simulink model "car_suspension_absolutedisplacements_BumpStops"  (R2024a)
settings: Solver=VariableStepAuto  StartTime=0.0  StopTime=5  RelTol=1e-3
values from neighbouring files (symbols this model uses):
  C1 = 800    [axle_params.mat]    (also in suspension_params.mat; task1.m = 700; task2.m; task3.m)
  C2 = 3000    [axle_params.mat]    (also in suspension_params.mat = 6000; task1.m = 1500; task2.m = 1500; task3.m = C2_vals(j))
  C3 = 200    [axle_params.mat]    (also in suspension_params.mat; task2.m; task3.m; task4.m)
  K1 = 2000    [axle_params.mat]    (also in suspension_params.mat; task1.m = 2200; task2.m; task3.m)
  K2 = 30000    [axle_params.mat]    (also in suspension_params.mat = 50000; task1.m = 13000; task2.m = 13000; task3.m = K2_vals(i))
  K3 = 100000    [axle_params.mat]    (also in suspension_params.mat; task1.m = 120000; task2.m; task3.m)
  M1 = 60    [axle_params.mat]    (also in suspension_params.mat; task1.m = 50; task2.m; task3.m)
  M2 = 250    [axle_params.mat]    (also in suspension_params.mat; task1.m; task2.m; task3.m)
  M3 = 100    [axle_params.mat]    (also in suspension_params.mat; task1.m; task2.m; task3.m)
settings Model: Creator=co1il  LastModifiedBy=Alex
settings SolverCC: AlgebraicLoopSolver=TrustRegion
settings DataIOCC: ReturnWorkspaceOutputs=off
settings DebuggingCC: UnconnectedInputMsg=warning  UnconnectedOutputMsg=warning  UnconnectedLineMsg=warning  PregeneratedLibrarySubsystemCodeDiagnostic=none  ArithmeticOperatorsInVariantConditions=warning
settings ModelReferenceCC: EnableRefExpFcnMdlSchedulingChecks=on
settings SFSimCC: SimUseLocalCustomCode=off  CustomCodeUndefinedFunction=UseInterfaceOnly
settings RTWCC: RTWUseLocalCustomCode=off  GPUComputeCapability=3.5
settings CodeAppCC: StateflowObjectComments=on

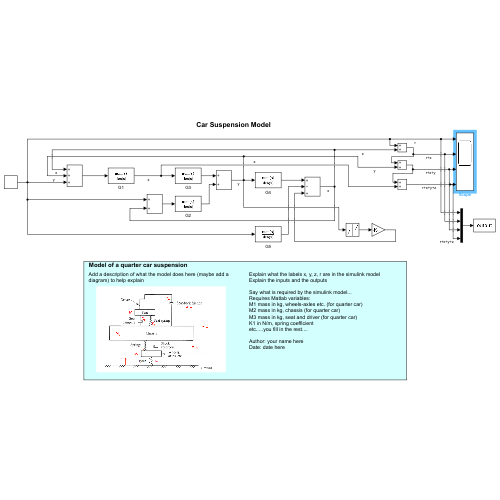
[thumbnail: Simulink's stored preview of the top-level diagram]
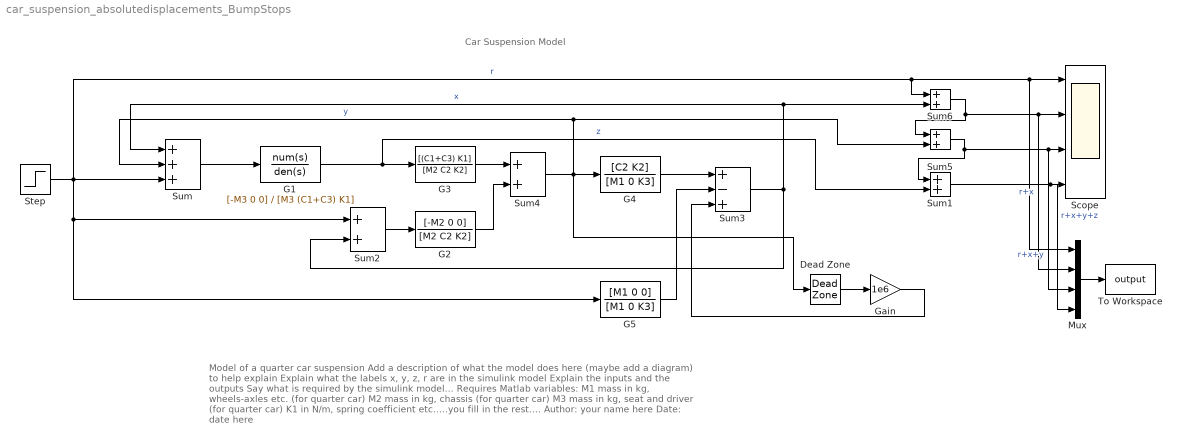
== system car_suspension_absolutedisplacements_BumpStops ==
  note: Model of a quarter car suspension
      |
      | Add a description of what the model does here (maybe add a diagram) to help explain
      |
      | Explain what the labels x, y, z, r are in the simulink model
      | Explain the inputs and the outputs
      |
      | Say what is required by the simulink model...
      | Requires Matlab variables:
      | M1 mass in kg, wheels-axles etc. (for quarter car)
      | M2 mass in kg, chassis (for quarter car)
      | M3 mass in kg, seat and driver (for quarter car)
      | K1 in N/m, spring coefficient
      | etc.....you fill in the rest....
      |
      | Author: your name here
      | Date: date here
  note: Car Suspension Model
  Dead Zone : DeadZone  LowerValue=-0.02  UpperValue=0.02
  G1 : TransferFcn  Numerator=[-M3 0 0]  Denominator=[M3 (C1+C3) K1]
  G2 : TransferFcn  Numerator=[-M2 0 0]  Denominator=[M2 C2 K2]
  G3 : TransferFcn  Numerator=[(C1+C3) K1]  Denominator=[M2 C2 K2]
  G4 : TransferFcn  Numerator=[C2 K2]  Denominator=[M1 0 K3]
  G5 : TransferFcn  Numerator=[M1 0 0]  Denominator=[M1 0 K3]
  Gain : Gain  Gain=1e6
  Mux : Mux
  Scope : Scope  NumInputPorts=4
  Step : Step  After=0.1  SampleTime=0
  Sum : Sum  Inputs=+++
  Sum{1..2,4..6} (5 alike) : Sum
  Sum3 : Sum  Inputs=+-+
  To Workspace : ToWorkspace  VariableName=output  SaveFormat=Timeseries  SampleTime=-1
  wires:
  G1/1 -> Sum1/2, G3/1  "z"
  Sum4/1 -> Dead Zone/1, Sum/2, Sum5/2, G4/1  "y"
  Sum/1 -> G1/1
  Sum3/1 -> Sum6/2, Sum/1, Sum2/2  "x"
  Sum2/1 -> G2/1
  G4/1 -> Sum3/1
  G5/1 -> Sum3/2
  G2/1 -> Sum4/2
  G3/1 -> Sum4/1
  Step/1 -> Sum6/1, Mux/1, Scope/1, Sum2/1, G5/1, Sum/3  "r"
  Mux/1 -> To Workspace/1
  Sum1/1 -> Mux/4, Scope/4  "r+x+y+z"
  Sum6/1 -> Mux/2, Scope/2, Sum5/1  "r+x"
  Sum5/1 -> Sum1/1, Mux/3, Scope/3  "r+x+y"
  Dead Zone/1 -> Gain/1
  Gain/1 -> Sum3/3
